simulink model "teststateflow"  (R2017a)
settings: Solver=VariableStepAuto  StartTime=0.0  StopTime=10.0  RelTol=1e-3
settings Model: Creator=Peter Vanhoef  LastModifiedBy=Peter Vanhoef

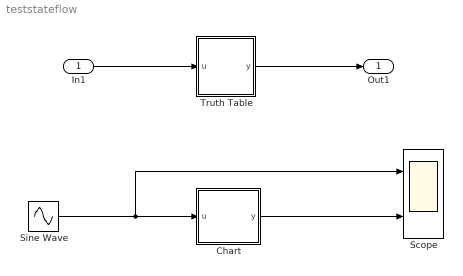
== system teststateflow ==
  In1 : Inport
  Chart : Stateflow chart  TreatAsAtomicUnit=on
  Scope : Scope  NumInputPorts=2
  Sine Wave : Sin  SampleTime=0
  Truth Table : Truth Table  TreatAsAtomicUnit=on
  Out1 : Outport
  wires:
  In1/1 -> Truth Table/1(u)
  Truth Table/1(y) -> Out1/1
  Sine Wave/1 -> Scope/1, Chart/1(u)
  Chart/1(y) -> Scope/2

== matlab function teststateflow/Truth Table ==
  data: u input; y output
function y = fcn(u)

aVarTruthTableCondition_1 = false;
aVarTruthTableCondition_2 = false;


% Example condition 1

aVarTruthTableCondition_1 = logical(u >= 0);

% Example condition 2

aVarTruthTableCondition_2 = logical(u ^ 2 <= 3);

if (aVarTruthTableCondition_1 && aVarTruthTableCondition_2)
    aFcnTruthTableAction_1();
elseif (~aVarTruthTableCondition_1 && aVarTruthTableCondition_2)
    aFcnTruthTableAction_1();
else % Default
    aFcnTruthTableAction_2();
end

function aFcnTruthTableAction_1()

% Example action 1 called from D1 & D2 column in condition table

y = u;

function aFcnTruthTableAction_2()

% Example action 2 called from D3 column in condition table

y = 1 / u;

== stateflow chart teststateflow/Chart ==
  state ON
    entry: y=1
  state OFF
    entry: y = -1
  (default) -> ON
  ON -> OFF : [u<0]
  OFF -> ON : [u>0]
  data: u input; y output
